simulink model "PSS_library"  (R2019b)
settings: Solver=VariableStepAuto  StartTime=0.0  StopTime=10.0  RelTol=1e-3
undefined symbols (not defined in the file or in its folder): dyn
libraries: modelLibrary x19
settings Model: Creator=gdudgeon  LastModifiedBy=gdudgeon
settings SFSimCC: CustomCodeUndefinedFunction=UseInterfaceOnly

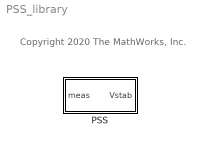
== system PSS_library ==
  note: Copyright 2020 The MathWorks, Inc.
  PSS : Subsystem  VariantControlMode=Label  Variant=on  LabelModeActiveChoice=Variant2
      settings: AttributesFormatString=%<BlockChoice>

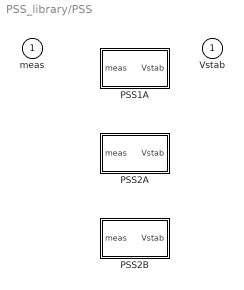
== system PSS_library/PSS ==
  meas : Inport
  PSS1A : Subsystem  VariantControl=Variant1  mask{p=dyn.pss1a_102_HYDRO}
      mask prompts: p "Parameters"
      mask DialogControl DescGroupVar Prompt: PSS1A
  PSS2A : Subsystem  VariantControl=Variant2  mask{p=dyn.pss2a_102_GAS}
      mask prompts: p "Parameters"
      mask DialogControl DescGroupVar Prompt: PSS2A
  PSS2B : Subsystem  VariantControl=Variant3  mask{p=dyn.pss2b_102_STEAM}
      mask prompts: p "Parameters"
      mask DialogControl DescGroupVar Prompt: PSS2B
  Vstab : Outport  VectorParamsAs1DForOutWhenUnconnected=off

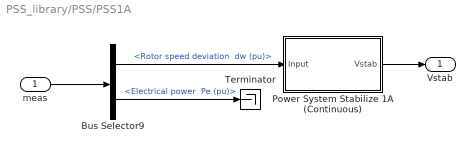
== system PSS_library/PSS/PSS1A ==
  meas : Inport
  Bus Selector9 : BusSelector  OutputSignals="Mechanical.Rotor speed deviation  dw (pu),Mechanical.Electrical power  Pe (pu)"
  Power System Stabilize 1A (Continuous) : Subsystem  mask(PSS1A - Single Input Power System Stabilizer){A1=p.a1, A2=p.a2, T1=p.t1, T2=p.t2, T3=p.t3, T4=p.t4, T5=p.t5, T6=p.t6, Ks=p.ks, Vrmax=p.vrmax, Vrmin=p.vrmin}
      mask prompts: A1 "A1, Notch filter parameter"; A2 "A2, Notch filter parameter"; T1 "T1, Lead/lag time constant [s]"; T2 "T2, Lead/lag time constant [s]"; T3 "T3, Lead/lag time constant [s]"; T4 "T4, Lead/lag time constant [s]"; T5 "T5, Washout time constant [s]"; T6 "T6, Transducer time constant [s]"; Ks "Ks, Stabilizer gain"; Vrmax "Vrmax, Maximum stabilizer output [pu]"; Vrmin "Vrmin, Minimize stabilizer output [pu]"
      mask DialogControl Container9 Prompt: Filter Time Constants
      mask DialogControl Container11 Prompt: Stabilizer
      mask Display:
      | port_label('input',1,'Input');
      | port_label('output',1,'Vstab');
      | 
      | color('blue');disp('PSS1A')
  Terminator : Terminator
  Vstab : Outport  VectorParamsAs1DForOutWhenUnconnected=off
  wires:
  meas/1 -> Bus Selector9/1
  Power System Stabilize 1A (Continuous)/1(Vstab) -> Vstab/1
  Bus Selector9/1 -> Power System Stabilize 1A (Continuous)/1(Input)  "<Rotor speed deviation  dw (pu)>"
  Bus Selector9/2 -> Terminator/1  "<Electrical power  Pe (pu)>"

== system PSS_library/PSS/PSS2A ==
  meas : Inport
  Bus Selector9 : BusSelector  OutputSignals="Mechanical.Rotor speed  wm  (pu),Mechanical.Electrical power  Pe (pu)"
  "Power System Stabilizer 2A (Continuous) " : Subsystem  mask(PSS2A - Duel Input Power System Stabilizer){TwSig1=[p.tw1 p.tw2], TwSig2=[p.tw3 p.tw4], T12=[p.t1 p.t2], T34=[p.t3 p.t4], T6=p.t6, T7=p.t7, T89=[p.t8 p.t9], Order=[p.n p.m], Tab=[p.a p.ta p.tb], Ks1=p.ks1, KsVec=[p.ks2 p.ks3 p.ks4], Vstmax=p.vstmax, Vstmin=p.vstmin}
      mask prompts: TwSig1 "[Tw1 Tw2], Washout Parameters, Signal #1"; TwSig2 "[Tw3 Tw4], Washout Parameters, Signal #2 [s]"; T12 "[T1 T2], Lead/lag time constant [s]"; T34 "[T3 T4], Lead/lag time constant [s]"; T6 "T6, Time Constant, Signal #1 [s]"; T7 "T7, Time Constant, Signal #2 [s]"; T89 "[T8 T9], Lead/Lag Ramp Tracking"; Order "[n m], Order of Tracking Filter"; Tab "[a Ta Tb], Gain/Lead/Lag Time Constants"; Ks1 "Ks1, Stabilizer Gain"; KsVec "[Ks2 Ks3 Ks4], Signal #2 Gains"; Vstmax "Vstmax, Maximum stabilizer output [pu]"; Vstmin "Vstmin, Minimize stabilizer output [pu]"
      mask init:
      | Tw1 = TwSig1(1);    Tw2 = TwSig1(2);
      | Tw3 = TwSig2(1);    Tw4 = TwSig2(2);
      | T1 = T12(1);        T2 = T12(2);
      | T3 = T34(1);        T4 = T34(2);
      | T8 = T89(1);        T9 = T89(2);
      | N = Order(1);       M = Order(2);
      | a = Tab(1);         Ta = Tab(2);        Tb = Tab(3);
      | Ks2 = KsVec(1);     Ks3 = KsVec(2);     Ks4 = KsVec(3);
      mask DialogControl Container9 Prompt: Filter Time Constants
      mask DialogControl Container11 Prompt: Stabilizer
      mask Display:
      | port_label('input',1,'Input 1');
      | port_label('input',2,'Input 2');
      | port_label('output',1,'Vstab');
      | 
      | color('blue');disp('PSS2A')
  Vstab : Outport  VectorParamsAs1DForOutWhenUnconnected=off
  wires:
  Bus Selector9/2 -> "Power System Stabilizer 2A (Continuous) "/2(Input_2)  "<Electrical power  Pe (pu)>"
  Bus Selector9/1 -> "Power System Stabilizer 2A (Continuous) "/1(Input_1)  "<Rotor speed  wm  (pu)>"
  "Power System Stabilizer 2A (Continuous) "/1(Vstab) -> Vstab/1
  meas/1 -> Bus Selector9/1

== system PSS_library/PSS/PSS2B ==
  meas : Inport
  Bus Selector3 : BusSelector  OutputSignals="Mechanical.Rotor speed deviation  dw (pu),Mechanical.Electrical power  Pe (pu)"
  "Power System Stabilizer 2B (Continuous) " : Subsystem  mask(PSS2A - Duel Input Power System Stabilizer){TwSig1=[p.tw1 p.tw2], TwSig2=[p.tw3 p.tw4], T12=[p.t1 p.t2], T34=[p.t3 p.t4], T6=p.t6, T7=p.t7, T89=[p.t8 p.t9], Order=[p.n p.m], Tab=[p.a p.ta p.tb], Ks1=p.ks1, KsVec=[p.ks2 p.ks3 p.ks4], Vstmax=p.vstmax, Vstmin=p.vstmin}
      mask prompts: TwSig1 "[Tw1 Tw2], Washout Parameters, Signal #1"; TwSig2 "[Tw3 Tw4], Washout Parameters, Signal #2 [s]"; T12 "[T1 T2], Lead/lag time constant [s]"; T34 "[T3 T4], Lead/lag time constant [s]"; T6 "T6, Time Constant, Signal #1 [s]"; T7 "T7, Time Constant, Signal #2 [s]"; T89 "[T8 T9], Lead/Lag Ramp Tracking"; Order "[n m], Order of Tracking Filter"; Tab "[a Ta Tb], Gain/Lead/Lag Time Constants"; Ks1 "Ks1, Stabilizer Gain"; KsVec "[Ks2 Ks3 Ks4], Signal #2 Gains"; Vstmax "Vstmax, Maximum stabilizer output [pu]"; Vstmin "Vstmin, Minimize stabilizer output [pu]"
      mask init: same as PSS_library/PSS/PSS2A/Power System Stabilizer 2A (Continuous) 
      mask DialogControl Container9 Prompt: Filter Time Constants
      mask DialogControl Container11 Prompt: Stabilizer
      mask Display:
      | port_label('input',1,'Input 1');
      | port_label('input',2,'Input 2');
      | port_label('output',1,'Vstab');
      | 
      | color('blue');disp('PSS2B')
  Vstab : Outport  VectorParamsAs1DForOutWhenUnconnected=off
  wires:
  "Power System Stabilizer 2B (Continuous) "/1(Vstab) -> Vstab/1
  meas/1 -> Bus Selector3/1
  Bus Selector3/1 -> "Power System Stabilizer 2B (Continuous) "/1(Input_1)  "<Rotor speed deviation  dw (pu)>"
  Bus Selector3/2 -> "Power System Stabilizer 2B (Continuous) "/2(Input_2)  "<Electrical power  Pe (pu)>"

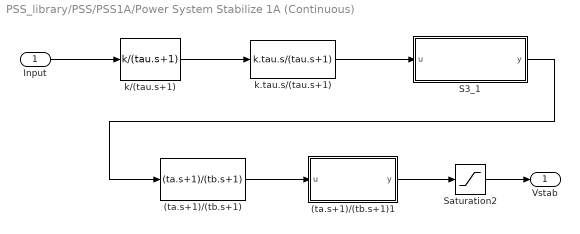
== system PSS_library/PSS/PSS1A/Power System Stabilize 1A (Continuous) ==
  Input : Inport
  (ta.s+1)/(tb.s+1) : modelLibrary/(ta.s+1)//(tb.s+1)  ta=T1  tb=T2
  (ta.s+1)/(tb.s+1)1 : Subsystem  mask{ta=T3, tb=T4}
      mask prompts: ta "numerator tau (ta)"; tb "denominator tau  (tb)"
  S3_1 : Subsystem
      mask Display: disp('1/(1+sA1 + s^2 A2)')
  Saturation2 : Saturate  UpperLimit=Vrmax  LowerLimit=Vrmin
      settings: AttributesFormatString=|
      | %<UpperLimit>
      | %<LowerLimit>
  k.tau.s/(tau.s+1) : modelLibrary/k.tau.s//(tau.s+1)  k=Ks  tau=T5
  k/(tau.s+1) : modelLibrary/k//(tau.s+1)  k=1  tau=T6  vmax=Inf  vmin=-Inf
  Vstab : Outport  VectorParamsAs1DForOutWhenUnconnected=off
  wires:
  Saturation2/1 -> Vstab/1
  (ta.s+1)/(tb.s+1)1/1(y) -> Saturation2/1
  (ta.s+1)/(tb.s+1)/1 -> (ta.s+1)/(tb.s+1)1/1(u)
  Input/1 -> k/(tau.s+1)/1
  k/(tau.s+1)/1 -> k.tau.s/(tau.s+1)/1
  S3_1/1(y) -> (ta.s+1)/(tb.s+1)/1
  k.tau.s/(tau.s+1)/1 -> S3_1/1(u)

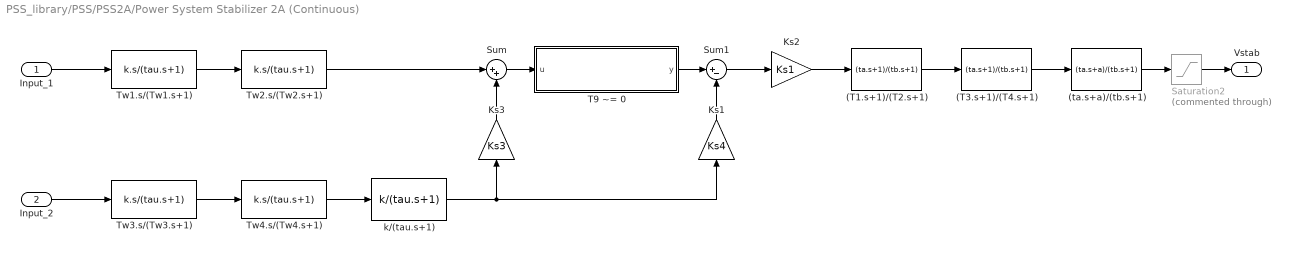
== system PSS_library/PSS/PSS2A/Power System Stabilizer 2A (Continuous)  ==
  Input_1 : Inport
  Input_2 : Inport  Port=2
  (T1.s+1)/(T2.s+1) : modelLibrary/(ta.s+1)//(tb.s+1)  ta=T1  tb=T2
  (T3.s+1)/(T4.s+1) : modelLibrary/(ta.s+1)//(tb.s+1)  ta=T3  tb=T4
  (ta.s+a)/(tb.s+1) : modelLibrary/(ta.s+a)//(tb.s+1)  ta=Ta  tb=Tb  a=a
  Ks1 : Gain  Gain=Ks4
  Ks2 : Gain  Gain=Ks1
  Ks3 : Gain  Gain=Ks3
  Saturation2 : Saturate  Commented=through  UpperLimit=Vstmax  LowerLimit=Vstmin
      settings: AttributesFormatString=|
      | %<UpperLimit>
      | %<LowerLimit>
  Sum : Sum  Inputs=|++
  Sum1 : Sum  Inputs=|+-
  T9 ~= 0 : Subsystem  VariantControl=T9NotZero  mask{M=M, N=N, T8=T8, T9=T9}
      mask prompts: M "M, Denominator Order"; N "N, Number of Series Filters"; T8 "T8, Lead Ramp Tracking Constant [s]"; T9 "T9, Lag Ramp Tracking Constant [s]"
      mask Display: disp('[(1 + s T_8) / (1 + s T_9)^m]^n','texmode','on');
  Tw1.s/(Tw1.s+1) : modelLibrary/k.s//(tau.s+1)  k=Tw1  tau=Tw1
  Tw2.s/(Tw2.s+1) : modelLibrary/k.s//(tau.s+1)  k=Tw2  tau=Tw2
  Tw3.s/(Tw3.s+1) : modelLibrary/k.s//(tau.s+1)  k=Tw3  tau=Tw3
  Tw4.s/(Tw4.s+1) : modelLibrary/k.s//(tau.s+1)  k=Tw4  tau=Tw4
  k/(tau.s+1) : modelLibrary/k//(tau.s+1)  k=Ks2  tau=T7  vmax=Inf  vmin=-Inf
  Vstab : Outport  VectorParamsAs1DForOutWhenUnconnected=off
  wires:
  (ta.s+a)/(tb.s+1)/1 -> Saturation2/1
  (T3.s+1)/(T4.s+1)/1 -> (ta.s+a)/(tb.s+1)/1
  (T1.s+1)/(T2.s+1)/1 -> (T3.s+1)/(T4.s+1)/1
  Ks2/1 -> (T1.s+1)/(T2.s+1)/1
  Saturation2/1 -> Vstab/1
  T9 ~= 0/1(y) -> Sum1/1
  Sum/1 -> T9 ~= 0/1(u)
  Sum1/1 -> Ks2/1
  Ks1/1 -> Sum1/2
  Ks3/1 -> Sum/2
  k/(tau.s+1)/1 -> Ks3/1, Ks1/1
  Tw2.s/(Tw2.s+1)/1 -> Sum/1
  Tw1.s/(Tw1.s+1)/1 -> Tw2.s/(Tw2.s+1)/1
  Input_1/1 -> Tw1.s/(Tw1.s+1)/1
  Input_2/1 -> Tw3.s/(Tw3.s+1)/1
  Tw3.s/(Tw3.s+1)/1 -> Tw4.s/(Tw4.s+1)/1
  Tw4.s/(Tw4.s+1)/1 -> k/(tau.s+1)/1

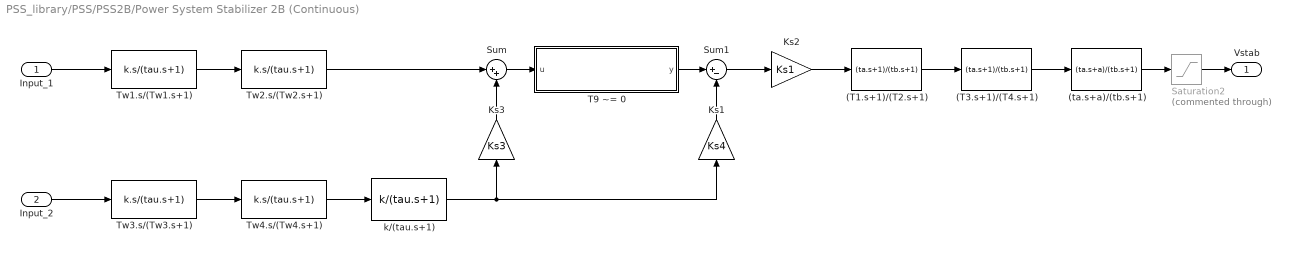
== system PSS_library/PSS/PSS2B/Power System Stabilizer 2B (Continuous)  ==
  Input_1 : Inport
  Input_2 : Inport  Port=2
  (T1.s+1)/(T2.s+1) : modelLibrary/(ta.s+1)//(tb.s+1)  ta=T1  tb=T2
  (T3.s+1)/(T4.s+1) : modelLibrary/(ta.s+1)//(tb.s+1)  ta=T3  tb=T4
  (ta.s+a)/(tb.s+1) : modelLibrary/(ta.s+a)//(tb.s+1)  ta=Ta  tb=Tb  a=a
  Ks1 : Gain  Gain=Ks4
  Ks2 : Gain  Gain=Ks1
  Ks3 : Gain  Gain=Ks3
  Saturation2 : Saturate  Commented=through  UpperLimit=Vstmax  LowerLimit=Vstmin
      settings: AttributesFormatString=|
      | %<UpperLimit>
      | %<LowerLimit>
  Sum : Sum  Inputs=|++
  Sum1 : Sum  Inputs=|+-
  T9 ~= 0 : Subsystem  VariantControl=T9NotZero  mask{M=M, N=N, T8=T8, T9=T9}
      mask prompts: M "M, Denominator Order"; N "N, Number of Series Filters"; T8 "T8, Lead Ramp Tracking Constant [s]"; T9 "T9, Lag Ramp Tracking Constant [s]"
      mask Display: disp('[(1 + s T_8) / (1 + s T_9)^m]^n','texmode','on');
  Tw1.s/(Tw1.s+1) : modelLibrary/k.s//(tau.s+1)  k=Tw1  tau=Tw1
  Tw2.s/(Tw2.s+1) : modelLibrary/k.s//(tau.s+1)  k=Tw2  tau=Tw2
  Tw3.s/(Tw3.s+1) : modelLibrary/k.s//(tau.s+1)  k=Tw3  tau=Tw3
  Tw4.s/(Tw4.s+1) : modelLibrary/k.s//(tau.s+1)  k=Tw4  tau=Tw4
  k/(tau.s+1) : modelLibrary/k//(tau.s+1)  k=Ks2  tau=T7  vmax=Inf  vmin=-Inf
  Vstab : Outport  VectorParamsAs1DForOutWhenUnconnected=off
  wires:
  (ta.s+a)/(tb.s+1)/1 -> Saturation2/1
  (T3.s+1)/(T4.s+1)/1 -> (ta.s+a)/(tb.s+1)/1
  (T1.s+1)/(T2.s+1)/1 -> (T3.s+1)/(T4.s+1)/1
  Ks2/1 -> (T1.s+1)/(T2.s+1)/1
  Saturation2/1 -> Vstab/1
  T9 ~= 0/1(y) -> Sum1/1
  Sum/1 -> T9 ~= 0/1(u)
  Sum1/1 -> Ks2/1
  Ks1/1 -> Sum1/2
  Ks3/1 -> Sum/2
  k/(tau.s+1)/1 -> Ks3/1, Ks1/1
  Tw2.s/(Tw2.s+1)/1 -> Sum/1
  Tw1.s/(Tw1.s+1)/1 -> Tw2.s/(Tw2.s+1)/1
  Input_1/1 -> Tw1.s/(Tw1.s+1)/1
  Input_2/1 -> Tw3.s/(Tw3.s+1)/1
  Tw3.s/(Tw3.s+1)/1 -> Tw4.s/(Tw4.s+1)/1
  Tw4.s/(Tw4.s+1)/1 -> k/(tau.s+1)/1

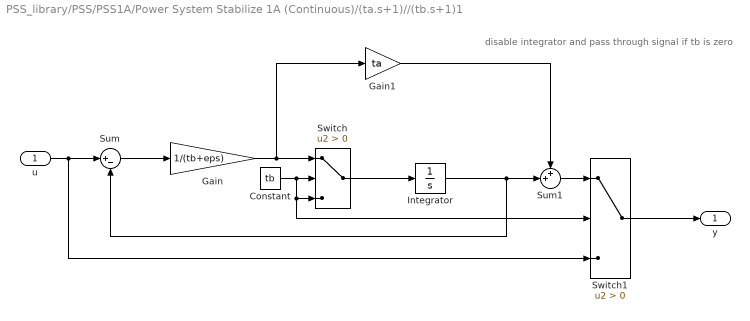
== system PSS_library/PSS/PSS1A/Power System Stabilize 1A (Continuous)/(ta.s+1)//(tb.s+1)1 ==
  note: disable integrator and pass through signal if tb is zero
  u : Inport
  Constant : Constant  Value=tb
  Gain : Gain  Gain=1/(tb+eps)
  Gain1 : Gain  Gain=ta
  Integrator : Integrator
  Sum : Sum  Inputs=|+-
  Sum1 : Sum  Inputs=++|
  Switch : Switch  Criteria=u2 > Threshold
  Switch1 : Switch  Criteria=u2 > Threshold
  y : Outport  VectorParamsAs1DForOutWhenUnconnected=off
  wires:
  Sum/1 -> Gain/1
  Gain/1 -> Switch/1, Gain1/1
  Gain1/1 -> Sum1/1
  Integrator/1 -> Sum1/2, Sum/2
  u/1 -> Switch1/3, Sum/1
  Constant/1 -> Switch1/2, Switch/3, Switch/2
  Switch/1 -> Integrator/1
  Sum1/1 -> Switch1/1
  Switch1/1 -> y/1

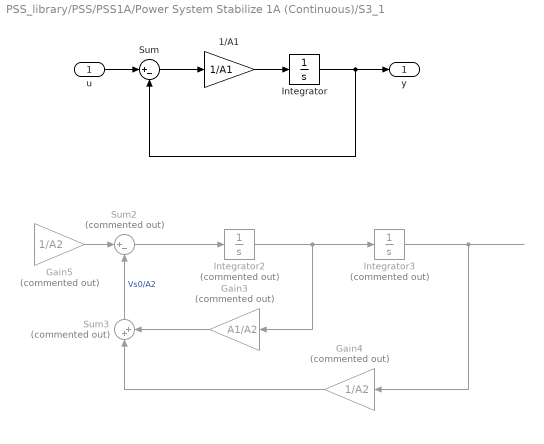
== system PSS_library/PSS/PSS1A/Power System Stabilize 1A (Continuous)/S3_1 ==
  u : Inport
  1/A1 : Gain  Gain=1/A1
  Gain3 : Gain  Commented=on  Gain=A1/A2
  Gain4 : Gain  Commented=on  Gain=1/A2
  Gain5 : Gain  Commented=on  Gain=1/A2
  Integrator : Integrator
  Integrator2 : Integrator  Commented=on
  Integrator3 : Integrator  Commented=on
  Sum : Sum  Inputs=|+-
  Sum2 : Sum  Commented=on  Inputs=|+-
  Sum3 : Sum  Commented=on  Inputs=|++
  y : Outport  InitialOutput=0  VectorParamsAs1DForOutWhenUnconnected=off
  wires:
  ? -> Gain5/1
  Integrator3/1 -> Gain4/1
  Integrator2/1 -> Integrator3/1, Gain3/1
  Sum2/1 -> Integrator2/1
  Gain5/1 -> Sum2/1
  Sum3/1 -> Sum2/2  "Vs0/A2"
  Gain3/1 -> Sum3/2
  Gain4/1 -> Sum3/1
  Sum/1 -> 1/A1/1
  1/A1/1 -> Integrator/1
  u/1 -> Sum/1
  Integrator/1 -> y/1, Sum/2

== system PSS_library/PSS/PSS2A/Power System Stabilizer 2A (Continuous) /T9 ~= 0 ==
  u : Inport
  Filter1 : Subsystem
      mask Display: disp('(1 + s T_8) / (1 + s T_9)^m','texmode','on');
  y : Outport  VectorParamsAs1DForOutWhenUnconnected=off
  wires:
  Filter1/1(Out1) -> y/1
  u/1 -> Filter1/1(In1)

== system PSS_library/PSS/PSS2B/Power System Stabilizer 2B (Continuous) /T9 ~= 0 ==
  u : Inport
  Filter1 : Subsystem
      mask Display: disp('(1 + s T_8) / (1 + s T_9)^m','texmode','on');
  y : Outport  VectorParamsAs1DForOutWhenUnconnected=off
  wires:
  Filter1/1(Out1) -> y/1
  u/1 -> Filter1/1(In1)

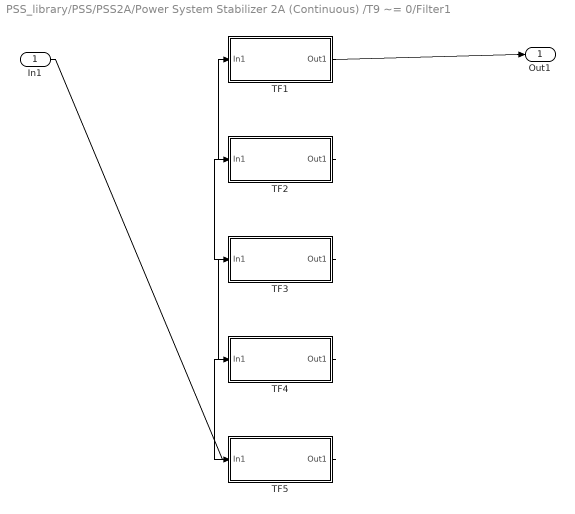
== system PSS_library/PSS/PSS2A/Power System Stabilizer 2A (Continuous) /T9 ~= 0/Filter1 ==
  In1 : Inport
  TF1 : Subsystem
      mask Display: disp('(1 + s T_8) / (1 + s T_9)','texmode','on');
  TF2 : Subsystem
      mask Display: disp('1 / (1 + s T_9)','texmode','on');
  TF3 : Subsystem
      mask Display: disp('1 / (1 + s T_9)','texmode','on');
  TF4 : Subsystem
      mask Display: disp('1 / (1 + s T_9)','texmode','on');
  TF5 : Subsystem
      mask Display: disp('1 / (1 + s T_9)','texmode','on');
  Out1 : Outport  VectorParamsAs1DForOutWhenUnconnected=off
  wires:
  TF1/1(Out1) -> Out1/1
  TF2/1(Out1) -> TF1/1(In1)
  TF3/1(Out1) -> TF2/1(In1)
  TF4/1(Out1) -> TF3/1(In1)
  TF5/1(Out1) -> TF4/1(In1)
  In1/1 -> TF5/1(In1)

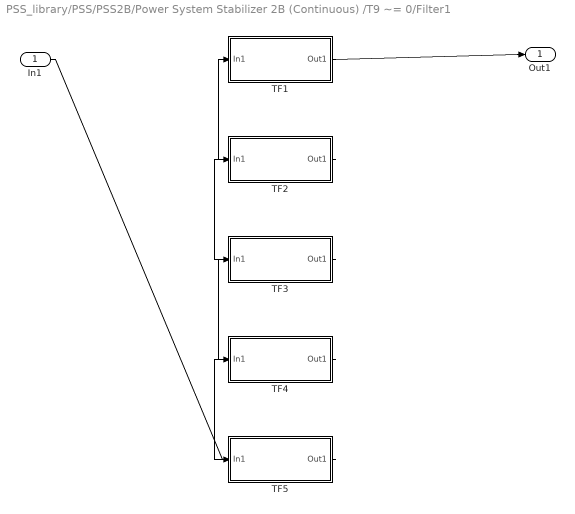
== system PSS_library/PSS/PSS2B/Power System Stabilizer 2B (Continuous) /T9 ~= 0/Filter1 ==
  In1 : Inport
  TF1 : Subsystem
      mask Display: disp('(1 + s T_8) / (1 + s T_9)','texmode','on');
  TF2 : Subsystem
      mask Display: disp('1 / (1 + s T_9)','texmode','on');
  TF3 : Subsystem
      mask Display: disp('1 / (1 + s T_9)','texmode','on');
  TF4 : Subsystem
      mask Display: disp('1 / (1 + s T_9)','texmode','on');
  TF5 : Subsystem
      mask Display: disp('1 / (1 + s T_9)','texmode','on');
  Out1 : Outport  VectorParamsAs1DForOutWhenUnconnected=off
  wires:
  TF1/1(Out1) -> Out1/1
  TF2/1(Out1) -> TF1/1(In1)
  TF3/1(Out1) -> TF2/1(In1)
  TF4/1(Out1) -> TF3/1(In1)
  TF5/1(Out1) -> TF4/1(In1)
  In1/1 -> TF5/1(In1)

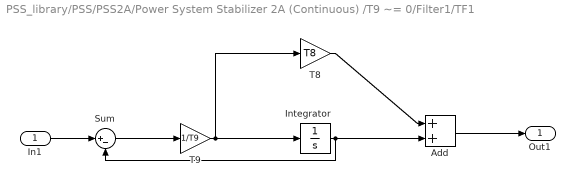
== system PSS_library/PSS/PSS2A/Power System Stabilizer 2A (Continuous) /T9 ~= 0/Filter1/TF1 ==
  In1 : Inport
  Add : Sum
  Integrator : Integrator
  Sum : Sum  Inputs=|+-
  T8 : Gain  Gain=T8
  T9 : Gain  Gain=1/T9
  Out1 : Outport  VectorParamsAs1DForOutWhenUnconnected=off
  wires:
  In1/1 -> Sum/1
  Sum/1 -> T9/1
  T9/1 -> Integrator/1, T8/1
  Integrator/1 -> Sum/2, Add/2
  T8/1 -> Add/1
  Add/1 -> Out1/1

== system PSS_library/PSS/PSS2A/Power System Stabilizer 2A (Continuous) /T9 ~= 0/Filter1/TF2 ==
  In1 : Inport
  Integrator : Integrator
  Sum : Sum  Inputs=|+-
  T9 : Gain  Gain=1/T9
  Out1 : Outport  VectorParamsAs1DForOutWhenUnconnected=off
  wires:
  In1/1 -> Sum/1
  Sum/1 -> T9/1
  T9/1 -> Integrator/1
  Integrator/1 -> Sum/2, Out1/1

== system PSS_library/PSS/PSS2A/Power System Stabilizer 2A (Continuous) /T9 ~= 0/Filter1/TF3 ==
  In1 : Inport
  Integrator : Integrator
  Sum : Sum  Inputs=|+-
  T9 : Gain  Gain=1/T9
  Out1 : Outport  VectorParamsAs1DForOutWhenUnconnected=off
  wires:
  In1/1 -> Sum/1
  Sum/1 -> T9/1
  T9/1 -> Integrator/1
  Integrator/1 -> Sum/2, Out1/1

== system PSS_library/PSS/PSS2A/Power System Stabilizer 2A (Continuous) /T9 ~= 0/Filter1/TF4 ==
  In1 : Inport
  Integrator : Integrator
  Sum : Sum  Inputs=|+-
  T9 : Gain  Gain=1/T9
  Out1 : Outport  VectorParamsAs1DForOutWhenUnconnected=off
  wires:
  In1/1 -> Sum/1
  Sum/1 -> T9/1
  T9/1 -> Integrator/1
  Integrator/1 -> Sum/2, Out1/1

== system PSS_library/PSS/PSS2A/Power System Stabilizer 2A (Continuous) /T9 ~= 0/Filter1/TF5 ==
  In1 : Inport
  Integrator : Integrator
  Sum : Sum  Inputs=|+-
  T9 : Gain  Gain=1/T9
  Out1 : Outport  VectorParamsAs1DForOutWhenUnconnected=off
  wires:
  In1/1 -> Sum/1
  Sum/1 -> T9/1
  T9/1 -> Integrator/1
  Integrator/1 -> Sum/2, Out1/1

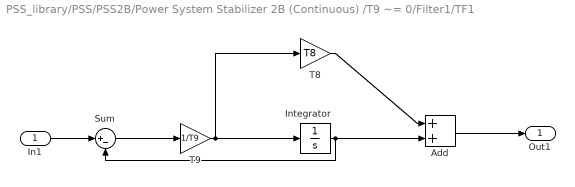
== system PSS_library/PSS/PSS2B/Power System Stabilizer 2B (Continuous) /T9 ~= 0/Filter1/TF1 ==
  In1 : Inport
  Add : Sum
  Integrator : Integrator
  Sum : Sum  Inputs=|+-
  T8 : Gain  Gain=T8
  T9 : Gain  Gain=1/T9
  Out1 : Outport  VectorParamsAs1DForOutWhenUnconnected=off
  wires:
  In1/1 -> Sum/1
  Sum/1 -> T9/1
  T9/1 -> Integrator/1, T8/1
  Integrator/1 -> Sum/2, Add/2
  T8/1 -> Add/1
  Add/1 -> Out1/1

== system PSS_library/PSS/PSS2B/Power System Stabilizer 2B (Continuous) /T9 ~= 0/Filter1/TF2 ==
  In1 : Inport
  Integrator : Integrator
  Sum : Sum  Inputs=|+-
  T9 : Gain  Gain=1/T9
  Out1 : Outport  VectorParamsAs1DForOutWhenUnconnected=off
  wires:
  In1/1 -> Sum/1
  Sum/1 -> T9/1
  T9/1 -> Integrator/1
  Integrator/1 -> Sum/2, Out1/1

== system PSS_library/PSS/PSS2B/Power System Stabilizer 2B (Continuous) /T9 ~= 0/Filter1/TF3 ==
  In1 : Inport
  Integrator : Integrator
  Sum : Sum  Inputs=|+-
  T9 : Gain  Gain=1/T9
  Out1 : Outport  VectorParamsAs1DForOutWhenUnconnected=off
  wires:
  In1/1 -> Sum/1
  Sum/1 -> T9/1
  T9/1 -> Integrator/1
  Integrator/1 -> Sum/2, Out1/1

== system PSS_library/PSS/PSS2B/Power System Stabilizer 2B (Continuous) /T9 ~= 0/Filter1/TF4 ==
  In1 : Inport
  Integrator : Integrator
  Sum : Sum  Inputs=|+-
  T9 : Gain  Gain=1/T9
  Out1 : Outport  VectorParamsAs1DForOutWhenUnconnected=off
  wires:
  In1/1 -> Sum/1
  Sum/1 -> T9/1
  T9/1 -> Integrator/1
  Integrator/1 -> Sum/2, Out1/1

== system PSS_library/PSS/PSS2B/Power System Stabilizer 2B (Continuous) /T9 ~= 0/Filter1/TF5 ==
  In1 : Inport
  Integrator : Integrator
  Sum : Sum  Inputs=|+-
  T9 : Gain  Gain=1/T9
  Out1 : Outport  VectorParamsAs1DForOutWhenUnconnected=off
  wires:
  In1/1 -> Sum/1
  Sum/1 -> T9/1
  T9/1 -> Integrator/1
  Integrator/1 -> Sum/2, Out1/1
